simulink model "quad_simulation_gen_data"  (R2020b)
settings: Solver=FixedStepAuto  StartTime=0.0  StopTime=20  FixedStep=0.01  RelTol=1e-3
settings Model: Creator=Duong  LastModifiedBy=ThinkPad
settings DataIOCC: ExternalInput=noise_freq
settings SFSimCC: CustomCodeUndefinedFunction=UseInterfaceOnly

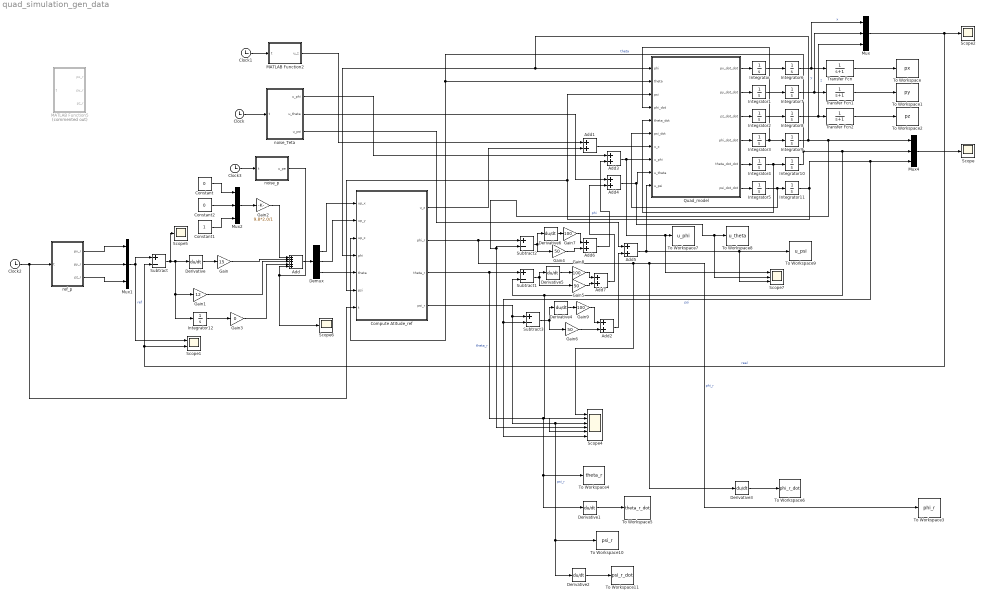
== system quad_simulation_gen_data ==
  Add : Sum  Inputs=+++++
  Add{1..7} (7 alike) : Sum
  Clock{,1..3} (4 alike) : Clock
  "Compute Atitude_ref " : MATLAB Function  TreatAsAtomicUnit=on
  Constant : Constant  Value=0
  Constant1 : Constant
  Constant2 : Constant  Value=0
  Demux : Demux  Outputs=3
  Derivative{,1..6} (7 alike) : Derivative
  Gain : Gain  Gain=15
  Gain1 : Gain  Gain=12
  Gain2 : Gain  Gain=9.8*2.0/1
  Gain3 : Gain  Gain=0
  Gain4 : Gain  Gain=50
  Gain5 : Gain  Gain=50
  Gain6 : Gain  Gain=50
  Gain7 : Gain  Gain=100
  Gain8 : Gain  Gain=100
  Gain9 : Gain  Gain=100
  Integrator{,1..5,7,9..12} (11 alike) : Integrator
  Integrator6 : Integrator  InitialCondition=2
  Integrator8 : Integrator  InitialCondition=-1
  MATLAB Function2 : MATLAB Function  TreatAsAtomicUnit=on
  MATLAB Function5 : MATLAB Function  Commented=on  TreatAsAtomicUnit=on
  Mux{,1..2,4} (4 alike) : Mux  Inputs=3
  "Quad_model " : MATLAB Function  TreatAsAtomicUnit=on
  Scope{,2,5..6} (4 alike) : Scope
  Scope1 : Scope  NumInputPorts=2
  Scope4 : Scope  NumInputPorts=6
  Scope7 : Scope  NumInputPorts=3
  Subtract{,1..3} (4 alike) : Sum  Inputs=+-
  To Workspace : ToWorkspace  VariableName=px  SampleTime=-1
      settings: Save2DSignal=2-D array (concatenate along first dimension)
  To Workspace1 : ToWorkspace  VariableName=py  SampleTime=-1
      settings: Save2DSignal=2-D array (concatenate along first dimension)
  To Workspace10 : ToWorkspace  VariableName=psi_r  SampleTime=-1
      settings: Save2DSignal=2-D array (concatenate along first dimension)
  To Workspace11 : ToWorkspace  VariableName=psi_r_dot  SampleTime=-1
      settings: Save2DSignal=2-D array (concatenate along first dimension)
  To Workspace2 : ToWorkspace  VariableName=pz  SampleTime=-1
      settings: Save2DSignal=2-D array (concatenate along first dimension)
  To Workspace3 : ToWorkspace  VariableName=phi_r  SampleTime=-1
      settings: Save2DSignal=2-D array (concatenate along first dimension)
  To Workspace4 : ToWorkspace  VariableName=theta_r  SampleTime=-1
      settings: Save2DSignal=2-D array (concatenate along first dimension)
  To Workspace5 : ToWorkspace  VariableName=theta_r_dot  SampleTime=-1
      settings: Save2DSignal=2-D array (concatenate along first dimension)
  To Workspace6 : ToWorkspace  VariableName=phi_r_dot  SampleTime=-1
      settings: Save2DSignal=2-D array (concatenate along first dimension)
  To Workspace7 : ToWorkspace  VariableName=u_phi  SampleTime=-1
      settings: Save2DSignal=2-D array (concatenate along first dimension)
  To Workspace8 : ToWorkspace  VariableName=u_theta  SampleTime=-1
      settings: Save2DSignal=2-D array (concatenate along first dimension)
  To Workspace9 : ToWorkspace  VariableName=u_psi  SampleTime=-1
      settings: Save2DSignal=2-D array (concatenate along first dimension)
  Transfer Fcn : TransferFcn  Denominator=[1 1]
  Transfer Fcn1 : TransferFcn  Denominator=[1 1]
  Transfer Fcn2 : TransferFcn  Denominator=[1 1]
  "noise_Teta " : MATLAB Function  TreatAsAtomicUnit=on
  "noise_p " : MATLAB Function  TreatAsAtomicUnit=on
  "ref_p " : MATLAB Function  TreatAsAtomicUnit=on
  wires:
  "Quad_model "/1(px_dot_dot) -> Integrator/1
  "Quad_model "/2(py_dot_dot) -> Integrator1/1
  "Quad_model "/3(pz_dot_dot) -> Integrator2/1
  "Quad_model "/4(phi_dot_dot) -> Integrator3/1
  "Quad_model "/5(theta_dot_dot) -> Integrator4/1
  "Quad_model "/6(psi_dot_dot) -> Integrator5/1
  Integrator/1 -> Integrator6/1
  Integrator1/1 -> Integrator7/1
  Integrator2/1 -> Integrator8/1
  Integrator3/1 -> Integrator9/1, "Quad_model "/4(phi_dot)
  Integrator4/1 -> Integrator10/1, "Quad_model "/5(theta_dot)
  Integrator5/1 -> "Quad_model "/6(psi_dot), Integrator11/1
  Integrator9/1 -> Subtract2/2, Scope4/4, Mux4/1, "Quad_model "/1(phi), "Compute Atitude_ref "/4(phi)  "phi"
  Integrator10/1 -> "Quad_model "/2(theta), "Compute Atitude_ref "/5(theta), Scope4/5, Subtract1/2, Mux4/2  "theta"
  Integrator11/1 -> Scope4/6, Subtract3/2, Mux4/3, "Quad_model "/3(psi), "Compute Atitude_ref "/6(psi)  "psi"
  Integrator6/1 -> Mux/1, Transfer Fcn/1  "x"
  Transfer Fcn/1 -> To Workspace/1
  Integrator7/1 -> Mux/2, Transfer Fcn1/1  "y"
  Transfer Fcn1/1 -> To Workspace1/1
  Integrator8/1 -> Mux/3, Transfer Fcn2/1  "z"
  Transfer Fcn2/1 -> To Workspace2/1
  Clock/1 -> "noise_Teta "/1(t)
  Clock1/1 -> MATLAB Function2/1(t)
  Add/1 -> Demux/1
  Mux/1 -> Scope1/2, Subtract/2, Scope2/1  "real"
  Mux1/1 -> Scope1/1, Subtract/1  "ref"
  Gain/1 -> Add/2
  Mux2/1 -> Gain2/1
  Derivative/1 -> Gain/1
  Gain2/1 -> Add/1
  Gain1/1 -> Add/3
  Constant1/1 -> Mux2/3
  Constant2/1 -> Mux2/2
  Constant/1 -> Mux2/1
  Subtract/1 -> Scope5/1, Integrator12/1, Gain1/1, Derivative/1
  Demux/1 -> "Compute Atitude_ref "/1(up_x)
  Demux/2 -> "Compute Atitude_ref "/2(up_y)
  Demux/3 -> "Compute Atitude_ref "/3(up_z)
  Mux4/1 -> Scope/1
  "Compute Atitude_ref "/3(theta_r) -> Subtract1/1, To Workspace4/1, Derivative1/1, Scope4/2  "theta_r"
  Subtract1/1 -> Gain5/1, Derivative5/1
  "Compute Atitude_ref "/2(phi_r) -> Scope4/1, To Workspace3/1, Derivative3/1, Subtract2/1  "phi_r"
  Subtract2/1 -> Gain4/1, Derivative6/1
  Subtract3/1 -> Gain6/1, Derivative4/1
  "Compute Atitude_ref "/4(psi_r) -> Derivative2/1, To Workspace10/1, Scope4/3, Subtract3/1  "psi_r"
  Integrator12/1 -> Gain3/1
  Gain3/1 -> Add/4
  Add1/1 -> "Quad_model "/7(u_z)
  "Compute Atitude_ref "/1(u_z) -> Add1/2
  MATLAB Function2/1(u_z) -> Add1/1
  "noise_Teta "/1(u_phi) -> Add3/1
  Add6/1 -> Add3/2
  Add3/1 -> "Quad_model "/8(u_phi), Scope7/1, To Workspace7/1
  Add7/1 -> Add4/2
  "noise_Teta "/2(u_theta) -> Add4/1
  Add4/1 -> Scope7/2, To Workspace8/1, "Quad_model "/9(u_theta)
  "noise_Teta "/3(u_psi) -> Add5/1
  Add2/1 -> Add5/2
  Add5/1 -> "Quad_model "/10(u_psi), Scope7/3, To Workspace9/1
  Derivative3/1 -> To Workspace6/1
  Derivative1/1 -> To Workspace5/1
  Clock2/1 -> "Compute Atitude_ref "/7(t), "ref_p "/1(t)
  "ref_p "/1(px_r) -> Mux1/1
  "ref_p "/2(py_r) -> Mux1/2
  "ref_p "/3(pz_r) -> Mux1/3
  Clock3/1 -> "noise_p "/1(t)
  "noise_p "/1(u_pe) -> Scope6/1, Add/5
  Derivative2/1 -> To Workspace11/1
  Derivative6/1 -> Gain7/1
  Derivative5/1 -> Gain8/1
  Derivative4/1 -> Gain9/1
  Gain9/1 -> Add2/1
  Gain6/1 -> Add2/2
  Gain8/1 -> Add7/1
  Gain5/1 -> Add7/2
  Gain7/1 -> Add6/1
  Gain4/1 -> Add6/2

== matlab function quad_simulation_gen_data/noise_Teta  ==
  data: t input; u_phi output; u_theta output; u_psi output
function [u_phi,u_theta,u_psi] = fcn(t)
noise_freq = zeros(3,1000);
noise_g = load('noise.mat');
noise_freq = noise_g.noise_freq;
freqNum = size(noise_freq,2);
u_noise = zeros(3,1);
for idx=1:freqNum
    u_noise = u_noise + 0*sin(noise_freq(:,idx)*t);
end
u_phi=u_noise(1);
u_theta=u_noise(2);
u_psi=u_noise(3);

== matlab function quad_simulation_gen_data/Quad_model  ==
  data: phi input; theta input; px_dot_dot output; py_dot_dot output; pz_dot_dot output; phi_dot_dot output; theta_dot_dot output; psi_dot_dot output; psi input; phi_dot input; theta_dot input; psi_dot input; u_z input; u_phi input; u_theta input; u_psi input
function [px_dot_dot, py_dot_dot, pz_dot_dot, phi_dot_dot, theta_dot_dot, psi_dot_dot] = fcn(phi,theta,psi,phi_dot,theta_dot,psi_dot,u_z,u_phi,u_theta,u_psi)
p_dot_dot=[0;0;0];
teta_dot_dot=[0;0;0];
px_dot_dot=0; py_dot_dot=0; pz_dot_dot=0;
phi_dot_dot=0; theta_dot_dot=0; psi_dot_dot=0;
m=2.0;
J=diag([5.1,5.1,10.2]);
k_w=1;
k_t=1;
g=9.8;
l_to=0.2;
J_theta=5.1; J_phi=5.1; J_psi=10.2;
u_teta=[u_phi;u_theta;u_psi];
R=[cos(theta)*cos(psi) (cos(psi)*sin(phi)*sin(theta)-cos(phi)*sin(psi)) (sin(phi)*sin(psi)+cos(phi)*cos(psi)*sin(theta));
    cos(theta)*sin(psi) (cos(phi)*cos(psi)+sin(phi)*sin(theta)*sin(psi)) (cos(phi)*sin(theta)*sin(psi)-cos(psi)*sin(phi));
-sin(theta) (cos(theta)*sin(phi)) (cos(phi)*cos(theta))];
%position dynamic
p_dot_dot=(1/m)*k_w*u_z*R*[0;0;1]-g*[0;0;1];
px_dot_dot=p_dot_dot(1);
py_dot_dot=p_dot_dot(2);
pz_dot_dot=p_dot_dot(3);
c11=0;
c12=(J_theta-J_psi)*(theta_dot*cos(phi)*sin(phi)+psi_dot*sin(phi)^2*cos(theta))/J_phi+((J_psi-J_theta)*psi_dot*cos(phi)^2*cos(theta)-J_phi*psi_dot*cos(theta))/J_phi;
c13=(J_psi-J_theta)*psi_dot*cos(phi)*sin(phi)*cos(theta)^2/J_phi;
c21=(J_psi-J_theta)*(theta_dot*cos(phi)*sin(phi)+psi_dot*sin(phi)^2*cos(theta))/J_theta+((J_theta-J_psi)*psi_dot*cos(phi)^2*cos(theta)+J_phi*psi_dot*cos(theta))/J_theta;
c22=(J_psi-J_theta)*phi_dot*cos(phi)*sin(phi)/J_theta;
c23=(-J_phi*psi_dot*sin(theta)*cos(theta)+J_psi*psi_dot*cos(phi)^2*cos(theta)*sin(theta))/J_theta+psi_dot*sin(phi)^2*cos(theta)*sin(theta);
c31=((J_theta-J_psi)*psi_dot*cos(theta)^2*sin(phi)*cos(phi)-J_phi*theta_dot*cos(theta))/J_psi;
c32=(J_psi-J_theta)*(theta_dot*cos(phi)*sin(phi)*sin(theta)+phi_dot*sin(phi)^2*cos(theta))/J_psi+((J_theta-J_psi)*phi_dot*cos(phi)^2*cos(theta)+J_phi*psi_dot*sin(theta)*cos(theta))/J_psi-J_theta*psi_dot*sin(phi)^2*sin(theta)*cos(theta)/J_psi-psi_dot*cos(phi)^2*cos(theta)*sin(theta);
c33=(-J_psi*theta_dot*cos(phi)^2*sin(theta)*cos(theta)-J_theta*theta_dot*sin(phi)^2*cos(theta)*sin(theta))/J_psi+((J_theta-J_psi)*phi_dot*cos(phi)*sin(phi)*cos(theta)^2+J_phi*theta_dot*sin(theta)*cos(theta))/J_psi;
C=[c11 c12 c13;
    c21 c22 c23;
    c31 c32 c33];
teta_dot=[phi_dot;theta_dot;psi_dot];
B=inv(J)*diag([(l_to*k_w),(l_to*k_w),(k_t)]);
teta_dot_dot=-inv(J)*C*teta_dot+B*u_teta;
phi_dot_dot=teta_dot_dot(1);
theta_dot_dot=teta_dot_dot(2);
psi_dot_dot=teta_dot_dot(3);

== matlab function quad_simulation_gen_data/MATLAB Function2 ==
  data: t input; u_z output
function u_z = fcn(t)

u_z = sum(0.1*sin([1 3 7 11 13 15]*t));
u_z = 0;

% if(t<2)
%     y=9.8*2/1+5;
% else y=9.8*2/1;
% end

== matlab function quad_simulation_gen_data/Compute Atitude_ref  ==
  settings: updateMethod=DISCRETE
  data: up_x input; up_y input; up_z input; u_z output; phi input; theta input; psi input; phi_r output; theta_r output; psi_r output; t input
function [u_z, phi_r, theta_r, psi_r] = fcn(up_x,up_y,up_z,phi,theta,psi,t)
u_z=up_z/(cos(theta)*cos(phi));
phi_r=asin((up_x*sin(psi) - up_y*cos(psi))/u_z);
theta_r=asin((up_x*cos(psi) + up_y*sin(psi))/(u_z*cos(phi)));
% phi_r=asin((cos(phi)*sin(theta)*sin(psi)-up_y/up_z)/cos(psi));
% theta_r=asin((up_x/u_z-sin(phi)*sin(psi))/(cos(psi)*cos(phi)));
psi_r=(0.4*sin(pi*t)+sum(0.01*sin(10*[rand(1) rand(1) rand(1) rand(1) rand(1)]*t)))*2^(-0.1*t);
psi_r=0;

== matlab function quad_simulation_gen_data/ref_p  ==
  data: t input; px_r output; py_r output; pz_r output
function [px_r,py_r,pz_r] = fcn(t)
f=0.1;
px_r = 2*sin(2*pi*f*t);
py_r = 2*cos(2*pi*f*t);
pz_r = 0.8*t;

== matlab function quad_simulation_gen_data/noise_p  ==
  data: t input; u_pe output
function u_pe = fcn(t)
a=0.2;
u_pe=zeros(3,1);
u_pex = sum(a*sin([1 3 7 11 13 15 27 29 98 99]*t));
u_pey = sum(a*sin([1 3 7 11 13 15 27 29 98 99]*t));
u_pez = sum(a*sin([1 3 7 11 13 15 27 29 98 99]*t));
u_pe=0*[u_pex;
    u_pey;
    u_pez];


% if(t<2)
%     y=9.8*2/1+5;
% else y=9.8*2/1;
% end

== matlab function quad_simulation_gen_data/MATLAB Function5 ==
  data: t input; px_r output; py_r output; pz_r output
function [px_r,py_r,pz_r] = fcn(t)
a = 0.1;
px_r  = 6*sin(a*t);
py_r = 6*sin(a*t);
pz_r = 0.8*t;
